simulink model "sm_car_display_battery_model"  (R2021a)
settings: Solver=VariableStepAuto  StartTime=0.0  StopTime=10.0  RelTol=1e-3
undefined symbols (not defined in the file or in its folder): X, Y, Z
libraries: sm_lib x98, nesl_utility x72, Cooling_Components x1
(part 2 of 4)

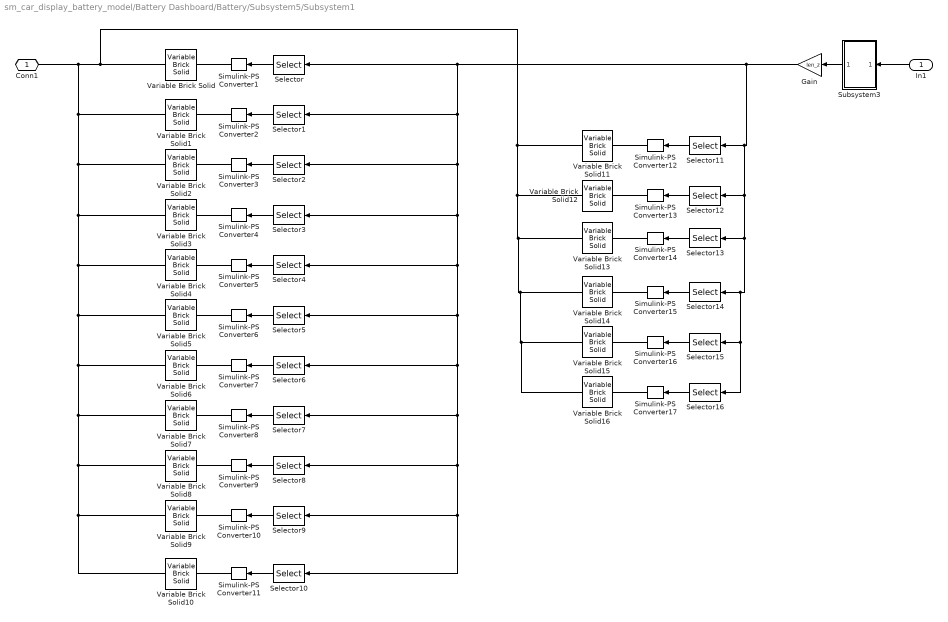
== system sm_car_display_battery_model/Battery Dashboard/Battery/Subsystem5/Subsystem1 ==
  In1 : Inport
  Gain : Gain  Gain=len_z
  Selector : Selector  InputPortWidth=numincr  IndexOptions=Index vector (dialog)  Indices=[1]  OutputSizes=1
  Selector1 : Selector  InputPortWidth=numincr  IndexOptions=Index vector (dialog)  Indices=[2]  OutputSizes=1
  Selector10 : Selector  InputPortWidth=numincr  IndexOptions=Index vector (dialog)  Indices=[11]  OutputSizes=1
  Selector11 : Selector  InputPortWidth=numincr  IndexOptions=Index vector (dialog)  Indices=[12]  OutputSizes=1
  Selector12 : Selector  InputPortWidth=numincr  IndexOptions=Index vector (dialog)  Indices=[13]  OutputSizes=1
  Selector13 : Selector  InputPortWidth=numincr  IndexOptions=Index vector (dialog)  Indices=[14]  OutputSizes=1
  Selector14 : Selector  InputPortWidth=numincr  IndexOptions=Index vector (dialog)  Indices=[15]  OutputSizes=1
  Selector15 : Selector  InputPortWidth=numincr  IndexOptions=Index vector (dialog)  Indices=[16]  OutputSizes=1
  Selector16 : Selector  InputPortWidth=numincr  IndexOptions=Index vector (dialog)  Indices=[17]  OutputSizes=1
  Selector2 : Selector  InputPortWidth=numincr  IndexOptions=Index vector (dialog)  Indices=[3]  OutputSizes=1
  Selector3 : Selector  InputPortWidth=numincr  IndexOptions=Index vector (dialog)  Indices=[4]  OutputSizes=1
  Selector4 : Selector  InputPortWidth=numincr  IndexOptions=Index vector (dialog)  Indices=[5]  OutputSizes=1
  Selector5 : Selector  InputPortWidth=numincr  IndexOptions=Index vector (dialog)  Indices=[6]  OutputSizes=1
  Selector6 : Selector  InputPortWidth=numincr  IndexOptions=Index vector (dialog)  Indices=[7]  OutputSizes=1
  Selector7 : Selector  InputPortWidth=numincr  IndexOptions=Index vector (dialog)  Indices=[8]  OutputSizes=1
  Selector8 : Selector  InputPortWidth=numincr  IndexOptions=Index vector (dialog)  Indices=[9]  OutputSizes=1
  Selector9 : Selector  InputPortWidth=numincr  IndexOptions=Index vector (dialog)  Indices=[10]  OutputSizes=1
  Simulink-PS Converter{1..17} (17 alike) : nesl_utility/Simulink-PS Converter  PhysicalDomain=network_engine_domain  SubClassName=ps_input  LeftPortType=input  RightPortType=output  PseudoPeriodic=off  Frequencies=[]  NoiseDistribution=none  NoiseParameters=[]  Unit=m  AffineConversion=off  FilteringAndDerivatives=provide  SimscapeFilterOrder=1  InputFilterTimeConstant=0.001  UdotUserProvided=0
      settings: SourceProductBaseCode=PW,SS
  Subsystem3 : Subsystem
  Variable Brick Solid : sm_lib/Body Elements/Variable Mass/Variable Brick Solid  XLengthType=Constant  XLength=len_x  XLengthUnits=m  YLengthType=Constant  YLength=len_y  YLengthUnits=m  ZLengthType=ProvidedByInput  ZLength=1  ZLengthUnits=m  MassType=CalculateFromGeometry  InitialMassType=Specified  InitialMass=1  InitialMassUnits=kg  Density=0.001  DensityUnits=kg/m^3  SenseXLength=off  SenseYLength=off  SenseZLength=off  SenseMass=off  SenseCenterOfMass=off  SenseInertiaMatrix=off  GraphicType=FromGeometry  MarkerShape=Sphere  MarkerSize=10  GraphicVisPropType=SimpleVisualProperties  GraphicDiffuseColor=[clr1]*17/numincr+[clr2]*0/numincr  GraphicSpecularColor=[0.5 0.5 0.5 1.0]  GraphicAmbientColor=[0.15 0.15 0.15 1.0]  GraphicEmissiveColor=[0.0 0.0 0.0 1.0]  GraphicShininess=75  GraphicOpacity=1.0
      settings: AttributesFormatString=%<GraphicDiffuseColor>  SourceProductBaseCode=MS
  Variable Brick Solid1 : sm_lib/Body Elements/Variable Mass/Variable Brick Solid  XLengthType=Constant  XLength=len_x  XLengthUnits=m  YLengthType=Constant  YLength=len_y  YLengthUnits=m  ZLengthType=ProvidedByInput  ZLength=1  ZLengthUnits=m  MassType=CalculateFromGeometry  InitialMassType=Specified  InitialMass=1  InitialMassUnits=kg  Density=0.001  DensityUnits=kg/m^3  SenseXLength=off  SenseYLength=off  SenseZLength=off  SenseMass=off  SenseCenterOfMass=off  SenseInertiaMatrix=off  GraphicType=FromGeometry  MarkerShape=Sphere  MarkerSize=10  GraphicVisPropType=SimpleVisualProperties  GraphicDiffuseColor=[clr1]*16/numincr+[clr2]*1/numincr  GraphicSpecularColor=[0.5 0.5 0.5 1.0]  GraphicAmbientColor=[0.15 0.15 0.15 1.0]  GraphicEmissiveColor=[0.0 0.0 0.0 1.0]  GraphicShininess=75  GraphicOpacity=1.0
      settings: AttributesFormatString=%<GraphicDiffuseColor>  SourceProductBaseCode=MS
  Variable Brick Solid10 : sm_lib/Body Elements/Variable Mass/Variable Brick Solid  XLengthType=Constant  XLength=len_x  XLengthUnits=m  YLengthType=Constant  YLength=len_y  YLengthUnits=m  ZLengthType=ProvidedByInput  ZLength=1  ZLengthUnits=m  MassType=CalculateFromGeometry  InitialMassType=Specified  InitialMass=1  InitialMassUnits=kg  Density=0.001  DensityUnits=kg/m^3  SenseXLength=off  SenseYLength=off  SenseZLength=off  SenseMass=off  SenseCenterOfMass=off  SenseInertiaMatrix=off  GraphicType=FromGeometry  MarkerShape=Sphere  MarkerSize=10  GraphicVisPropType=SimpleVisualProperties  GraphicDiffuseColor=[clr1]*7/numincr+[clr2]*10/numincr  GraphicSpecularColor=[0.5 0.5 0.5 1.0]  GraphicAmbientColor=[0.15 0.15 0.15 1.0]  GraphicEmissiveColor=[0.0 0.0 0.0 1.0]  GraphicShininess=75  GraphicOpacity=1.0
      settings: AttributesFormatString=%<GraphicDiffuseColor>  SourceProductBaseCode=MS
  Variable Brick Solid11 : sm_lib/Body Elements/Variable Mass/Variable Brick Solid  XLengthType=Constant  XLength=len_x  XLengthUnits=m  YLengthType=Constant  YLength=len_y  YLengthUnits=m  ZLengthType=ProvidedByInput  ZLength=1  ZLengthUnits=m  MassType=CalculateFromGeometry  InitialMassType=Specified  InitialMass=1  InitialMassUnits=kg  Density=0.001  DensityUnits=kg/m^3  SenseXLength=off  SenseYLength=off  SenseZLength=off  SenseMass=off  SenseCenterOfMass=off  SenseInertiaMatrix=off  GraphicType=FromGeometry  MarkerShape=Sphere  MarkerSize=10  GraphicVisPropType=SimpleVisualProperties  GraphicDiffuseColor=[clr1]*6/numincr+[clr2]*11/numincr  GraphicSpecularColor=[0.5 0.5 0.5 1.0]  GraphicAmbientColor=[0.15 0.15 0.15 1.0]  GraphicEmissiveColor=[0.0 0.0 0.0 1.0]  GraphicShininess=75  GraphicOpacity=1.0
      settings: AttributesFormatString=%<GraphicDiffuseColor>  SourceProductBaseCode=MS
  Variable Brick Solid12 : sm_lib/Body Elements/Variable Mass/Variable Brick Solid  XLengthType=Constant  XLength=len_x  XLengthUnits=m  YLengthType=Constant  YLength=len_y  YLengthUnits=m  ZLengthType=ProvidedByInput  ZLength=1  ZLengthUnits=m  MassType=CalculateFromGeometry  InitialMassType=Specified  InitialMass=1  InitialMassUnits=kg  Density=0.001  DensityUnits=kg/m^3  SenseXLength=off  SenseYLength=off  SenseZLength=off  SenseMass=off  SenseCenterOfMass=off  SenseInertiaMatrix=off  GraphicType=FromGeometry  MarkerShape=Sphere  MarkerSize=10  GraphicVisPropType=SimpleVisualProperties  GraphicDiffuseColor=[clr1]*5/numincr+[clr2]*12/numincr  GraphicSpecularColor=[0.5 0.5 0.5 1.0]  GraphicAmbientColor=[0.15 0.15 0.15 1.0]  GraphicEmissiveColor=[0.0 0.0 0.0 1.0]  GraphicShininess=75  GraphicOpacity=1.0
      settings: AttributesFormatString=%<GraphicDiffuseColor>  SourceProductBaseCode=MS
  Variable Brick Solid13 : sm_lib/Body Elements/Variable Mass/Variable Brick Solid  XLengthType=Constant  XLength=len_x  XLengthUnits=m  YLengthType=Constant  YLength=len_y  YLengthUnits=m  ZLengthType=ProvidedByInput  ZLength=1  ZLengthUnits=m  MassType=CalculateFromGeometry  InitialMassType=Specified  InitialMass=1  InitialMassUnits=kg  Density=0.001  DensityUnits=kg/m^3  SenseXLength=off  SenseYLength=off  SenseZLength=off  SenseMass=off  SenseCenterOfMass=off  SenseInertiaMatrix=off  GraphicType=FromGeometry  MarkerShape=Sphere  MarkerSize=10  GraphicVisPropType=SimpleVisualProperties  GraphicDiffuseColor=[clr1]*4/numincr+[clr2]*13/numincr  GraphicSpecularColor=[0.5 0.5 0.5 1.0]  GraphicAmbientColor=[0.15 0.15 0.15 1.0]  GraphicEmissiveColor=[0.0 0.0 0.0 1.0]  GraphicShininess=75  GraphicOpacity=1.0
      settings: AttributesFormatString=%<GraphicDiffuseColor>  SourceProductBaseCode=MS
  Variable Brick Solid14 : sm_lib/Body Elements/Variable Mass/Variable Brick Solid  XLengthType=Constant  XLength=len_x  XLengthUnits=m  YLengthType=Constant  YLength=len_y  YLengthUnits=m  ZLengthType=ProvidedByInput  ZLength=1  ZLengthUnits=m  MassType=CalculateFromGeometry  InitialMassType=Specified  InitialMass=1  InitialMassUnits=kg  Density=0.001  DensityUnits=kg/m^3  SenseXLength=off  SenseYLength=off  SenseZLength=off  SenseMass=off  SenseCenterOfMass=off  SenseInertiaMatrix=off  GraphicType=FromGeometry  MarkerShape=Sphere  MarkerSize=10  GraphicVisPropType=SimpleVisualProperties  GraphicDiffuseColor=[clr1]*3/numincr+[clr2]*14/numincr  GraphicSpecularColor=[0.5 0.5 0.5 1.0]  GraphicAmbientColor=[0.15 0.15 0.15 1.0]  GraphicEmissiveColor=[0.0 0.0 0.0 1.0]  GraphicShininess=75  GraphicOpacity=1.0
      settings: AttributesFormatString=%<GraphicDiffuseColor>  SourceProductBaseCode=MS
  Variable Brick Solid15 : sm_lib/Body Elements/Variable Mass/Variable Brick Solid  XLengthType=Constant  XLength=len_x  XLengthUnits=m  YLengthType=Constant  YLength=len_y  YLengthUnits=m  ZLengthType=ProvidedByInput  ZLength=1  ZLengthUnits=m  MassType=CalculateFromGeometry  InitialMassType=Specified  InitialMass=1  InitialMassUnits=kg  Density=0.001  DensityUnits=kg/m^3  SenseXLength=off  SenseYLength=off  SenseZLength=off  SenseMass=off  SenseCenterOfMass=off  SenseInertiaMatrix=off  GraphicType=FromGeometry  MarkerShape=Sphere  MarkerSize=10  GraphicVisPropType=SimpleVisualProperties  GraphicDiffuseColor=[clr1]*2/numincr+[clr2]*15/numincr  GraphicSpecularColor=[0.5 0.5 0.5 1.0]  GraphicAmbientColor=[0.15 0.15 0.15 1.0]  GraphicEmissiveColor=[0.0 0.0 0.0 1.0]  GraphicShininess=75  GraphicOpacity=1.0
      settings: AttributesFormatString=%<GraphicDiffuseColor>  SourceProductBaseCode=MS
  Variable Brick Solid16 : sm_lib/Body Elements/Variable Mass/Variable Brick Solid  XLengthType=Constant  XLength=len_x  XLengthUnits=m  YLengthType=Constant  YLength=len_y  YLengthUnits=m  ZLengthType=ProvidedByInput  ZLength=1  ZLengthUnits=m  MassType=CalculateFromGeometry  InitialMassType=Specified  InitialMass=1  InitialMassUnits=kg  Density=0.001  DensityUnits=kg/m^3  SenseXLength=off  SenseYLength=off  SenseZLength=off  SenseMass=off  SenseCenterOfMass=off  SenseInertiaMatrix=off  GraphicType=FromGeometry  MarkerShape=Sphere  MarkerSize=10  GraphicVisPropType=SimpleVisualProperties  GraphicDiffuseColor=[clr1]*1/numincr+[clr2]*16/numincr  GraphicSpecularColor=[0.5 0.5 0.5 1.0]  GraphicAmbientColor=[0.15 0.15 0.15 1.0]  GraphicEmissiveColor=[0.0 0.0 0.0 1.0]  GraphicShininess=75  GraphicOpacity=1.0
      settings: AttributesFormatString=%<GraphicDiffuseColor>  SourceProductBaseCode=MS
  Variable Brick Solid2 : sm_lib/Body Elements/Variable Mass/Variable Brick Solid  XLengthType=Constant  XLength=len_x  XLengthUnits=m  YLengthType=Constant  YLength=len_y  YLengthUnits=m  ZLengthType=ProvidedByInput  ZLength=1  ZLengthUnits=m  MassType=CalculateFromGeometry  InitialMassType=Specified  InitialMass=1  InitialMassUnits=kg  Density=0.001  DensityUnits=kg/m^3  SenseXLength=off  SenseYLength=off  SenseZLength=off  SenseMass=off  SenseCenterOfMass=off  SenseInertiaMatrix=off  GraphicType=FromGeometry  MarkerShape=Sphere  MarkerSize=10  GraphicVisPropType=SimpleVisualProperties  GraphicDiffuseColor=[clr1]*15/numincr+[clr2]*2/numincr  GraphicSpecularColor=[0.5 0.5 0.5 1.0]  GraphicAmbientColor=[0.15 0.15 0.15 1.0]  GraphicEmissiveColor=[0.0 0.0 0.0 1.0]  GraphicShininess=75  GraphicOpacity=1.0
      settings: AttributesFormatString=%<GraphicDiffuseColor>  SourceProductBaseCode=MS
  Variable Brick Solid3 : sm_lib/Body Elements/Variable Mass/Variable Brick Solid  XLengthType=Constant  XLength=len_x  XLengthUnits=m  YLengthType=Constant  YLength=len_y  YLengthUnits=m  ZLengthType=ProvidedByInput  ZLength=1  ZLengthUnits=m  MassType=CalculateFromGeometry  InitialMassType=Specified  InitialMass=1  InitialMassUnits=kg  Density=0.001  DensityUnits=kg/m^3  SenseXLength=off  SenseYLength=off  SenseZLength=off  SenseMass=off  SenseCenterOfMass=off  SenseInertiaMatrix=off  GraphicType=FromGeometry  MarkerShape=Sphere  MarkerSize=10  GraphicVisPropType=SimpleVisualProperties  GraphicDiffuseColor=[clr1]*14/numincr+[clr2]*3/numincr  GraphicSpecularColor=[0.5 0.5 0.5 1.0]  GraphicAmbientColor=[0.15 0.15 0.15 1.0]  GraphicEmissiveColor=[0.0 0.0 0.0 1.0]  GraphicShininess=75  GraphicOpacity=1.0
      settings: AttributesFormatString=%<GraphicDiffuseColor>  SourceProductBaseCode=MS
  Variable Brick Solid4 : sm_lib/Body Elements/Variable Mass/Variable Brick Solid  XLengthType=Constant  XLength=len_x  XLengthUnits=m  YLengthType=Constant  YLength=len_y  YLengthUnits=m  ZLengthType=ProvidedByInput  ZLength=1  ZLengthUnits=m  MassType=CalculateFromGeometry  InitialMassType=Specified  InitialMass=1  InitialMassUnits=kg  Density=0.001  DensityUnits=kg/m^3  SenseXLength=off  SenseYLength=off  SenseZLength=off  SenseMass=off  SenseCenterOfMass=off  SenseInertiaMatrix=off  GraphicType=FromGeometry  MarkerShape=Sphere  MarkerSize=10  GraphicVisPropType=SimpleVisualProperties  GraphicDiffuseColor=[clr1]*13/numincr+[clr2]*4/numincr  GraphicSpecularColor=[0.5 0.5 0.5 1.0]  GraphicAmbientColor=[0.15 0.15 0.15 1.0]  GraphicEmissiveColor=[0.0 0.0 0.0 1.0]  GraphicShininess=75  GraphicOpacity=1.0
      settings: AttributesFormatString=%<GraphicDiffuseColor>  SourceProductBaseCode=MS
  Variable Brick Solid5 : sm_lib/Body Elements/Variable Mass/Variable Brick Solid  XLengthType=Constant  XLength=len_x  XLengthUnits=m  YLengthType=Constant  YLength=len_y  YLengthUnits=m  ZLengthType=ProvidedByInput  ZLength=1  ZLengthUnits=m  MassType=CalculateFromGeometry  InitialMassType=Specified  InitialMass=1  InitialMassUnits=kg  Density=0.001  DensityUnits=kg/m^3  SenseXLength=off  SenseYLength=off  SenseZLength=off  SenseMass=off  SenseCenterOfMass=off  SenseInertiaMatrix=off  GraphicType=FromGeometry  MarkerShape=Sphere  MarkerSize=10  GraphicVisPropType=SimpleVisualProperties  GraphicDiffuseColor=[clr1]*12/numincr+[clr2]*5/numincr  GraphicSpecularColor=[0.5 0.5 0.5 1.0]  GraphicAmbientColor=[0.15 0.15 0.15 1.0]  GraphicEmissiveColor=[0.0 0.0 0.0 1.0]  GraphicShininess=75  GraphicOpacity=1.0
      settings: AttributesFormatString=%<GraphicDiffuseColor>  SourceProductBaseCode=MS
  Variable Brick Solid6 : sm_lib/Body Elements/Variable Mass/Variable Brick Solid  XLengthType=Constant  XLength=len_x  XLengthUnits=m  YLengthType=Constant  YLength=len_y  YLengthUnits=m  ZLengthType=ProvidedByInput  ZLength=1  ZLengthUnits=m  MassType=CalculateFromGeometry  InitialMassType=Specified  InitialMass=1  InitialMassUnits=kg  Density=0.001  DensityUnits=kg/m^3  SenseXLength=off  SenseYLength=off  SenseZLength=off  SenseMass=off  SenseCenterOfMass=off  SenseInertiaMatrix=off  GraphicType=FromGeometry  MarkerShape=Sphere  MarkerSize=10  GraphicVisPropType=SimpleVisualProperties  GraphicDiffuseColor=[clr1]*11/numincr+[clr2]*6/numincr  GraphicSpecularColor=[0.5 0.5 0.5 1.0]  GraphicAmbientColor=[0.15 0.15 0.15 1.0]  GraphicEmissiveColor=[0.0 0.0 0.0 1.0]  GraphicShininess=75  GraphicOpacity=1.0
      settings: AttributesFormatString=%<GraphicDiffuseColor>  SourceProductBaseCode=MS
  Variable Brick Solid7 : sm_lib/Body Elements/Variable Mass/Variable Brick Solid  XLengthType=Constant  XLength=len_x  XLengthUnits=m  YLengthType=Constant  YLength=len_y  YLengthUnits=m  ZLengthType=ProvidedByInput  ZLength=1  ZLengthUnits=m  MassType=CalculateFromGeometry  InitialMassType=Specified  InitialMass=1  InitialMassUnits=kg  Density=0.001  DensityUnits=kg/m^3  SenseXLength=off  SenseYLength=off  SenseZLength=off  SenseMass=off  SenseCenterOfMass=off  SenseInertiaMatrix=off  GraphicType=FromGeometry  MarkerShape=Sphere  MarkerSize=10  GraphicVisPropType=SimpleVisualProperties  GraphicDiffuseColor=[clr1]*10/numincr+[clr2]*7/numincr  GraphicSpecularColor=[0.5 0.5 0.5 1.0]  GraphicAmbientColor=[0.15 0.15 0.15 1.0]  GraphicEmissiveColor=[0.0 0.0 0.0 1.0]  GraphicShininess=75  GraphicOpacity=1.0
      settings: AttributesFormatString=%<GraphicDiffuseColor>  SourceProductBaseCode=MS
  Variable Brick Solid8 : sm_lib/Body Elements/Variable Mass/Variable Brick Solid  XLengthType=Constant  XLength=len_x  XLengthUnits=m  YLengthType=Constant  YLength=len_y  YLengthUnits=m  ZLengthType=ProvidedByInput  ZLength=1  ZLengthUnits=m  MassType=CalculateFromGeometry  InitialMassType=Specified  InitialMass=1  InitialMassUnits=kg  Density=0.001  DensityUnits=kg/m^3  SenseXLength=off  SenseYLength=off  SenseZLength=off  SenseMass=off  SenseCenterOfMass=off  SenseInertiaMatrix=off  GraphicType=FromGeometry  MarkerShape=Sphere  MarkerSize=10  GraphicVisPropType=SimpleVisualProperties  GraphicDiffuseColor=[clr1]*9/numincr+[clr2]*8/numincr  GraphicSpecularColor=[0.5 0.5 0.5 1.0]  GraphicAmbientColor=[0.15 0.15 0.15 1.0]  GraphicEmissiveColor=[0.0 0.0 0.0 1.0]  GraphicShininess=75  GraphicOpacity=1.0
      settings: AttributesFormatString=%<GraphicDiffuseColor>  SourceProductBaseCode=MS
  Variable Brick Solid9 : sm_lib/Body Elements/Variable Mass/Variable Brick Solid  XLengthType=Constant  XLength=len_x  XLengthUnits=m  YLengthType=Constant  YLength=len_y  YLengthUnits=m  ZLengthType=ProvidedByInput  ZLength=1  ZLengthUnits=m  MassType=CalculateFromGeometry  InitialMassType=Specified  InitialMass=1  InitialMassUnits=kg  Density=0.001  DensityUnits=kg/m^3  SenseXLength=off  SenseYLength=off  SenseZLength=off  SenseMass=off  SenseCenterOfMass=off  SenseInertiaMatrix=off  GraphicType=FromGeometry  MarkerShape=Sphere  MarkerSize=10  GraphicVisPropType=SimpleVisualProperties  GraphicDiffuseColor=[clr1]*8/numincr+[clr2]*9/numincr  GraphicSpecularColor=[0.5 0.5 0.5 1.0]  GraphicAmbientColor=[0.15 0.15 0.15 1.0]  GraphicEmissiveColor=[0.0 0.0 0.0 1.0]  GraphicShininess=75  GraphicOpacity=1.0
      settings: AttributesFormatString=%<GraphicDiffuseColor>  SourceProductBaseCode=MS
  Conn1 : PMIOPort  Side=Right
  wires:
  Selector/1 -> Simulink-PS Converter1/1
  Selector1/1 -> Simulink-PS Converter2/1
  Selector2/1 -> Simulink-PS Converter3/1
  Selector3/1 -> Simulink-PS Converter4/1
  Selector4/1 -> Simulink-PS Converter5/1
  Selector5/1 -> Simulink-PS Converter6/1
  Selector6/1 -> Simulink-PS Converter7/1
  Selector7/1 -> Simulink-PS Converter8/1
  Selector8/1 -> Simulink-PS Converter9/1
  Selector9/1 -> Simulink-PS Converter10/1
  Selector10/1 -> Simulink-PS Converter11/1
  Selector11/1 -> Simulink-PS Converter12/1
  Selector12/1 -> Simulink-PS Converter13/1
  Selector13/1 -> Simulink-PS Converter14/1
  Selector14/1 -> Simulink-PS Converter15/1
  Selector15/1 -> Simulink-PS Converter16/1
  In1/1 -> Subsystem3/1(In1)
  Selector16/1 -> Simulink-PS Converter17/1
  Gain/1 -> Selector16/1, Selector15/1, Selector14/1, Selector13/1, Selector12/1, Selector11/1, Selector10/1, Selector9/1, Selector8/1, Selector7/1, Selector6/1, Selector5/1, Selector4/1, Selector3/1, Selector2/1, Selector1/1, Selector/1
  Subsystem3/1(Out1) -> Gain/1
  connections:
  Simulink-PS Converter1/RConn1 -- Variable Brick Solid/LConn1
  Variable Brick Solid12/RConn1 -- Variable Brick Solid1/RConn1 -- Variable Brick Solid2/RConn1 -- Variable Brick Solid3/RConn1 -- Variable Brick Solid5/RConn1 -- Variable Brick Solid6/RConn1 -- Variable Brick Solid7/RConn1 -- Variable Brick Solid8/RConn1 -- Variable Brick Solid9/RConn1 -- Variable Brick Solid10/RConn1 -- Variable Brick Solid4/RConn1 -- Conn1/RConn1 -- Variable Brick Solid/RConn1 -- Variable Brick Solid11/RConn1 -- Variable Brick Solid13/RConn1 -- Variable Brick Solid14/RConn1 -- Variable Brick Solid15/RConn1 -- Variable Brick Solid16/RConn1
  Simulink-PS Converter2/RConn1 -- Variable Brick Solid1/LConn1
  Variable Brick Solid2/LConn1 -- Simulink-PS Converter3/RConn1
  Variable Brick Solid3/LConn1 -- Simulink-PS Converter4/RConn1
  Variable Brick Solid4/LConn1 -- Simulink-PS Converter5/RConn1
  Variable Brick Solid5/LConn1 -- Simulink-PS Converter6/RConn1
  Variable Brick Solid6/LConn1 -- Simulink-PS Converter7/RConn1
  Variable Brick Solid7/LConn1 -- Simulink-PS Converter8/RConn1
  Variable Brick Solid8/LConn1 -- Simulink-PS Converter9/RConn1
  Variable Brick Solid9/LConn1 -- Simulink-PS Converter10/RConn1
  Variable Brick Solid10/LConn1 -- Simulink-PS Converter11/RConn1
  Variable Brick Solid11/LConn1 -- Simulink-PS Converter12/RConn1
  Variable Brick Solid12/LConn1 -- Simulink-PS Converter13/RConn1
  Variable Brick Solid13/LConn1 -- Simulink-PS Converter14/RConn1
  Variable Brick Solid14/LConn1 -- Simulink-PS Converter15/RConn1
  Variable Brick Solid15/LConn1 -- Simulink-PS Converter16/RConn1
  Variable Brick Solid16/LConn1 -- Simulink-PS Converter17/RConn1

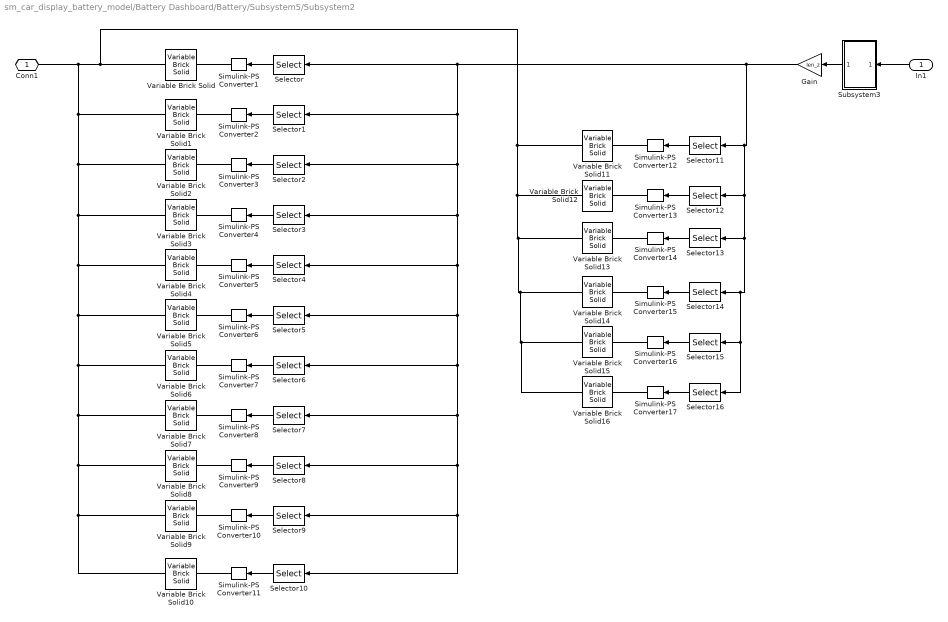
== system sm_car_display_battery_model/Battery Dashboard/Battery/Subsystem5/Subsystem2 ==
  In1 : Inport
  Gain : Gain  Gain=len_z
  Selector : Selector  InputPortWidth=numincr  IndexOptions=Index vector (dialog)  Indices=[1]  OutputSizes=1
  Selector1 : Selector  InputPortWidth=numincr  IndexOptions=Index vector (dialog)  Indices=[2]  OutputSizes=1
  Selector10 : Selector  InputPortWidth=numincr  IndexOptions=Index vector (dialog)  Indices=[11]  OutputSizes=1
  Selector11 : Selector  InputPortWidth=numincr  IndexOptions=Index vector (dialog)  Indices=[12]  OutputSizes=1
  Selector12 : Selector  InputPortWidth=numincr  IndexOptions=Index vector (dialog)  Indices=[13]  OutputSizes=1
  Selector13 : Selector  InputPortWidth=numincr  IndexOptions=Index vector (dialog)  Indices=[14]  OutputSizes=1
  Selector14 : Selector  InputPortWidth=numincr  IndexOptions=Index vector (dialog)  Indices=[15]  OutputSizes=1
  Selector15 : Selector  InputPortWidth=numincr  IndexOptions=Index vector (dialog)  Indices=[16]  OutputSizes=1
  Selector16 : Selector  InputPortWidth=numincr  IndexOptions=Index vector (dialog)  Indices=[17]  OutputSizes=1
  Selector2 : Selector  InputPortWidth=numincr  IndexOptions=Index vector (dialog)  Indices=[3]  OutputSizes=1
  Selector3 : Selector  InputPortWidth=numincr  IndexOptions=Index vector (dialog)  Indices=[4]  OutputSizes=1
  Selector4 : Selector  InputPortWidth=numincr  IndexOptions=Index vector (dialog)  Indices=[5]  OutputSizes=1
  Selector5 : Selector  InputPortWidth=numincr  IndexOptions=Index vector (dialog)  Indices=[6]  OutputSizes=1
  Selector6 : Selector  InputPortWidth=numincr  IndexOptions=Index vector (dialog)  Indices=[7]  OutputSizes=1
  Selector7 : Selector  InputPortWidth=numincr  IndexOptions=Index vector (dialog)  Indices=[8]  OutputSizes=1
  Selector8 : Selector  InputPortWidth=numincr  IndexOptions=Index vector (dialog)  Indices=[9]  OutputSizes=1
  Selector9 : Selector  InputPortWidth=numincr  IndexOptions=Index vector (dialog)  Indices=[10]  OutputSizes=1
  Simulink-PS Converter{1..17} (17 alike) : nesl_utility/Simulink-PS Converter  PhysicalDomain=network_engine_domain  SubClassName=ps_input  LeftPortType=input  RightPortType=output  PseudoPeriodic=off  Frequencies=[]  NoiseDistribution=none  NoiseParameters=[]  Unit=m  AffineConversion=off  FilteringAndDerivatives=provide  SimscapeFilterOrder=1  InputFilterTimeConstant=0.001  UdotUserProvided=0
      settings: SourceProductBaseCode=PW,SS
  Subsystem3 : Subsystem
  Variable Brick Solid : sm_lib/Body Elements/Variable Mass/Variable Brick Solid  XLengthType=Constant  XLength=len_x  XLengthUnits=m  YLengthType=Constant  YLength=len_y  YLengthUnits=m  ZLengthType=ProvidedByInput  ZLength=1  ZLengthUnits=m  MassType=CalculateFromGeometry  InitialMassType=Specified  InitialMass=1  InitialMassUnits=kg  Density=0.001  DensityUnits=kg/m^3  SenseXLength=off  SenseYLength=off  SenseZLength=off  SenseMass=off  SenseCenterOfMass=off  SenseInertiaMatrix=off  GraphicType=FromGeometry  MarkerShape=Sphere  MarkerSize=10  GraphicVisPropType=SimpleVisualProperties  GraphicDiffuseColor=[clr1]*17/numincr+[clr2]*0/numincr  GraphicSpecularColor=[0.5 0.5 0.5 1.0]  GraphicAmbientColor=[0.15 0.15 0.15 1.0]  GraphicEmissiveColor=[0.0 0.0 0.0 1.0]  GraphicShininess=75  GraphicOpacity=1.0
      settings: AttributesFormatString=%<GraphicDiffuseColor>  SourceProductBaseCode=MS
  Variable Brick Solid1 : sm_lib/Body Elements/Variable Mass/Variable Brick Solid  XLengthType=Constant  XLength=len_x  XLengthUnits=m  YLengthType=Constant  YLength=len_y  YLengthUnits=m  ZLengthType=ProvidedByInput  ZLength=1  ZLengthUnits=m  MassType=CalculateFromGeometry  InitialMassType=Specified  InitialMass=1  InitialMassUnits=kg  Density=0.001  DensityUnits=kg/m^3  SenseXLength=off  SenseYLength=off  SenseZLength=off  SenseMass=off  SenseCenterOfMass=off  SenseInertiaMatrix=off  GraphicType=FromGeometry  MarkerShape=Sphere  MarkerSize=10  GraphicVisPropType=SimpleVisualProperties  GraphicDiffuseColor=[clr1]*16/numincr+[clr2]*1/numincr  GraphicSpecularColor=[0.5 0.5 0.5 1.0]  GraphicAmbientColor=[0.15 0.15 0.15 1.0]  GraphicEmissiveColor=[0.0 0.0 0.0 1.0]  GraphicShininess=75  GraphicOpacity=1.0
      settings: AttributesFormatString=%<GraphicDiffuseColor>  SourceProductBaseCode=MS
  Variable Brick Solid10 : sm_lib/Body Elements/Variable Mass/Variable Brick Solid  XLengthType=Constant  XLength=len_x  XLengthUnits=m  YLengthType=Constant  YLength=len_y  YLengthUnits=m  ZLengthType=ProvidedByInput  ZLength=1  ZLengthUnits=m  MassType=CalculateFromGeometry  InitialMassType=Specified  InitialMass=1  InitialMassUnits=kg  Density=0.001  DensityUnits=kg/m^3  SenseXLength=off  SenseYLength=off  SenseZLength=off  SenseMass=off  SenseCenterOfMass=off  SenseInertiaMatrix=off  GraphicType=FromGeometry  MarkerShape=Sphere  MarkerSize=10  GraphicVisPropType=SimpleVisualProperties  GraphicDiffuseColor=[clr1]*7/numincr+[clr2]*10/numincr  GraphicSpecularColor=[0.5 0.5 0.5 1.0]  GraphicAmbientColor=[0.15 0.15 0.15 1.0]  GraphicEmissiveColor=[0.0 0.0 0.0 1.0]  GraphicShininess=75  GraphicOpacity=1.0
      settings: AttributesFormatString=%<GraphicDiffuseColor>  SourceProductBaseCode=MS
  Variable Brick Solid11 : sm_lib/Body Elements/Variable Mass/Variable Brick Solid  XLengthType=Constant  XLength=len_x  XLengthUnits=m  YLengthType=Constant  YLength=len_y  YLengthUnits=m  ZLengthType=ProvidedByInput  ZLength=1  ZLengthUnits=m  MassType=CalculateFromGeometry  InitialMassType=Specified  InitialMass=1  InitialMassUnits=kg  Density=0.001  DensityUnits=kg/m^3  SenseXLength=off  SenseYLength=off  SenseZLength=off  SenseMass=off  SenseCenterOfMass=off  SenseInertiaMatrix=off  GraphicType=FromGeometry  MarkerShape=Sphere  MarkerSize=10  GraphicVisPropType=SimpleVisualProperties  GraphicDiffuseColor=[clr1]*6/numincr+[clr2]*11/numincr  GraphicSpecularColor=[0.5 0.5 0.5 1.0]  GraphicAmbientColor=[0.15 0.15 0.15 1.0]  GraphicEmissiveColor=[0.0 0.0 0.0 1.0]  GraphicShininess=75  GraphicOpacity=1.0
      settings: AttributesFormatString=%<GraphicDiffuseColor>  SourceProductBaseCode=MS
  Variable Brick Solid12 : sm_lib/Body Elements/Variable Mass/Variable Brick Solid  XLengthType=Constant  XLength=len_x  XLengthUnits=m  YLengthType=Constant  YLength=len_y  YLengthUnits=m  ZLengthType=ProvidedByInput  ZLength=1  ZLengthUnits=m  MassType=CalculateFromGeometry  InitialMassType=Specified  InitialMass=1  InitialMassUnits=kg  Density=0.001  DensityUnits=kg/m^3  SenseXLength=off  SenseYLength=off  SenseZLength=off  SenseMass=off  SenseCenterOfMass=off  SenseInertiaMatrix=off  GraphicType=FromGeometry  MarkerShape=Sphere  MarkerSize=10  GraphicVisPropType=SimpleVisualProperties  GraphicDiffuseColor=[clr1]*5/numincr+[clr2]*12/numincr  GraphicSpecularColor=[0.5 0.5 0.5 1.0]  GraphicAmbientColor=[0.15 0.15 0.15 1.0]  GraphicEmissiveColor=[0.0 0.0 0.0 1.0]  GraphicShininess=75  GraphicOpacity=1.0
      settings: AttributesFormatString=%<GraphicDiffuseColor>  SourceProductBaseCode=MS
  Variable Brick Solid13 : sm_lib/Body Elements/Variable Mass/Variable Brick Solid  XLengthType=Constant  XLength=len_x  XLengthUnits=m  YLengthType=Constant  YLength=len_y  YLengthUnits=m  ZLengthType=ProvidedByInput  ZLength=1  ZLengthUnits=m  MassType=CalculateFromGeometry  InitialMassType=Specified  InitialMass=1  InitialMassUnits=kg  Density=0.001  DensityUnits=kg/m^3  SenseXLength=off  SenseYLength=off  SenseZLength=off  SenseMass=off  SenseCenterOfMass=off  SenseInertiaMatrix=off  GraphicType=FromGeometry  MarkerShape=Sphere  MarkerSize=10  GraphicVisPropType=SimpleVisualProperties  GraphicDiffuseColor=[clr1]*4/numincr+[clr2]*13/numincr  GraphicSpecularColor=[0.5 0.5 0.5 1.0]  GraphicAmbientColor=[0.15 0.15 0.15 1.0]  GraphicEmissiveColor=[0.0 0.0 0.0 1.0]  GraphicShininess=75  GraphicOpacity=1.0
      settings: AttributesFormatString=%<GraphicDiffuseColor>  SourceProductBaseCode=MS
  Variable Brick Solid14 : sm_lib/Body Elements/Variable Mass/Variable Brick Solid  XLengthType=Constant  XLength=len_x  XLengthUnits=m  YLengthType=Constant  YLength=len_y  YLengthUnits=m  ZLengthType=ProvidedByInput  ZLength=1  ZLengthUnits=m  MassType=CalculateFromGeometry  InitialMassType=Specified  InitialMass=1  InitialMassUnits=kg  Density=0.001  DensityUnits=kg/m^3  SenseXLength=off  SenseYLength=off  SenseZLength=off  SenseMass=off  SenseCenterOfMass=off  SenseInertiaMatrix=off  GraphicType=FromGeometry  MarkerShape=Sphere  MarkerSize=10  GraphicVisPropType=SimpleVisualProperties  GraphicDiffuseColor=[clr1]*3/numincr+[clr2]*14/numincr  GraphicSpecularColor=[0.5 0.5 0.5 1.0]  GraphicAmbientColor=[0.15 0.15 0.15 1.0]  GraphicEmissiveColor=[0.0 0.0 0.0 1.0]  GraphicShininess=75  GraphicOpacity=1.0
      settings: AttributesFormatString=%<GraphicDiffuseColor>  SourceProductBaseCode=MS
  Variable Brick Solid15 : sm_lib/Body Elements/Variable Mass/Variable Brick Solid  XLengthType=Constant  XLength=len_x  XLengthUnits=m  YLengthType=Constant  YLength=len_y  YLengthUnits=m  ZLengthType=ProvidedByInput  ZLength=1  ZLengthUnits=m  MassType=CalculateFromGeometry  InitialMassType=Specified  InitialMass=1  InitialMassUnits=kg  Density=0.001  DensityUnits=kg/m^3  SenseXLength=off  SenseYLength=off  SenseZLength=off  SenseMass=off  SenseCenterOfMass=off  SenseInertiaMatrix=off  GraphicType=FromGeometry  MarkerShape=Sphere  MarkerSize=10  GraphicVisPropType=SimpleVisualProperties  GraphicDiffuseColor=[clr1]*2/numincr+[clr2]*15/numincr  GraphicSpecularColor=[0.5 0.5 0.5 1.0]  GraphicAmbientColor=[0.15 0.15 0.15 1.0]  GraphicEmissiveColor=[0.0 0.0 0.0 1.0]  GraphicShininess=75  GraphicOpacity=1.0
      settings: AttributesFormatString=%<GraphicDiffuseColor>  SourceProductBaseCode=MS
  Variable Brick Solid16 : sm_lib/Body Elements/Variable Mass/Variable Brick Solid  XLengthType=Constant  XLength=len_x  XLengthUnits=m  YLengthType=Constant  YLength=len_y  YLengthUnits=m  ZLengthType=ProvidedByInput  ZLength=1  ZLengthUnits=m  MassType=CalculateFromGeometry  InitialMassType=Specified  InitialMass=1  InitialMassUnits=kg  Density=0.001  DensityUnits=kg/m^3  SenseXLength=off  SenseYLength=off  SenseZLength=off  SenseMass=off  SenseCenterOfMass=off  SenseInertiaMatrix=off  GraphicType=FromGeometry  MarkerShape=Sphere  MarkerSize=10  GraphicVisPropType=SimpleVisualProperties  GraphicDiffuseColor=[clr1]*1/numincr+[clr2]*16/numincr  GraphicSpecularColor=[0.5 0.5 0.5 1.0]  GraphicAmbientColor=[0.15 0.15 0.15 1.0]  GraphicEmissiveColor=[0.0 0.0 0.0 1.0]  GraphicShininess=75  GraphicOpacity=1.0
      settings: AttributesFormatString=%<GraphicDiffuseColor>  SourceProductBaseCode=MS
  Variable Brick Solid2 : sm_lib/Body Elements/Variable Mass/Variable Brick Solid  XLengthType=Constant  XLength=len_x  XLengthUnits=m  YLengthType=Constant  YLength=len_y  YLengthUnits=m  ZLengthType=ProvidedByInput  ZLength=1  ZLengthUnits=m  MassType=CalculateFromGeometry  InitialMassType=Specified  InitialMass=1  InitialMassUnits=kg  Density=0.001  DensityUnits=kg/m^3  SenseXLength=off  SenseYLength=off  SenseZLength=off  SenseMass=off  SenseCenterOfMass=off  SenseInertiaMatrix=off  GraphicType=FromGeometry  MarkerShape=Sphere  MarkerSize=10  GraphicVisPropType=SimpleVisualProperties  GraphicDiffuseColor=[clr1]*15/numincr+[clr2]*2/numincr  GraphicSpecularColor=[0.5 0.5 0.5 1.0]  GraphicAmbientColor=[0.15 0.15 0.15 1.0]  GraphicEmissiveColor=[0.0 0.0 0.0 1.0]  GraphicShininess=75  GraphicOpacity=1.0
      settings: AttributesFormatString=%<GraphicDiffuseColor>  SourceProductBaseCode=MS
  Variable Brick Solid3 : sm_lib/Body Elements/Variable Mass/Variable Brick Solid  XLengthType=Constant  XLength=len_x  XLengthUnits=m  YLengthType=Constant  YLength=len_y  YLengthUnits=m  ZLengthType=ProvidedByInput  ZLength=1  ZLengthUnits=m  MassType=CalculateFromGeometry  InitialMassType=Specified  InitialMass=1  InitialMassUnits=kg  Density=0.001  DensityUnits=kg/m^3  SenseXLength=off  SenseYLength=off  SenseZLength=off  SenseMass=off  SenseCenterOfMass=off  SenseInertiaMatrix=off  GraphicType=FromGeometry  MarkerShape=Sphere  MarkerSize=10  GraphicVisPropType=SimpleVisualProperties  GraphicDiffuseColor=[clr1]*14/numincr+[clr2]*3/numincr  GraphicSpecularColor=[0.5 0.5 0.5 1.0]  GraphicAmbientColor=[0.15 0.15 0.15 1.0]  GraphicEmissiveColor=[0.0 0.0 0.0 1.0]  GraphicShininess=75  GraphicOpacity=1.0
      settings: AttributesFormatString=%<GraphicDiffuseColor>  SourceProductBaseCode=MS
  Variable Brick Solid4 : sm_lib/Body Elements/Variable Mass/Variable Brick Solid  XLengthType=Constant  XLength=len_x  XLengthUnits=m  YLengthType=Constant  YLength=len_y  YLengthUnits=m  ZLengthType=ProvidedByInput  ZLength=1  ZLengthUnits=m  MassType=CalculateFromGeometry  InitialMassType=Specified  InitialMass=1  InitialMassUnits=kg  Density=0.001  DensityUnits=kg/m^3  SenseXLength=off  SenseYLength=off  SenseZLength=off  SenseMass=off  SenseCenterOfMass=off  SenseInertiaMatrix=off  GraphicType=FromGeometry  MarkerShape=Sphere  MarkerSize=10  GraphicVisPropType=SimpleVisualProperties  GraphicDiffuseColor=[clr1]*13/numincr+[clr2]*4/numincr  GraphicSpecularColor=[0.5 0.5 0.5 1.0]  GraphicAmbientColor=[0.15 0.15 0.15 1.0]  GraphicEmissiveColor=[0.0 0.0 0.0 1.0]  GraphicShininess=75  GraphicOpacity=1.0
      settings: AttributesFormatString=%<GraphicDiffuseColor>  SourceProductBaseCode=MS
  Variable Brick Solid5 : sm_lib/Body Elements/Variable Mass/Variable Brick Solid  XLengthType=Constant  XLength=len_x  XLengthUnits=m  YLengthType=Constant  YLength=len_y  YLengthUnits=m  ZLengthType=ProvidedByInput  ZLength=1  ZLengthUnits=m  MassType=CalculateFromGeometry  InitialMassType=Specified  InitialMass=1  InitialMassUnits=kg  Density=0.001  DensityUnits=kg/m^3  SenseXLength=off  SenseYLength=off  SenseZLength=off  SenseMass=off  SenseCenterOfMass=off  SenseInertiaMatrix=off  GraphicType=FromGeometry  MarkerShape=Sphere  MarkerSize=10  GraphicVisPropType=SimpleVisualProperties  GraphicDiffuseColor=[clr1]*12/numincr+[clr2]*5/numincr  GraphicSpecularColor=[0.5 0.5 0.5 1.0]  GraphicAmbientColor=[0.15 0.15 0.15 1.0]  GraphicEmissiveColor=[0.0 0.0 0.0 1.0]  GraphicShininess=75  GraphicOpacity=1.0
      settings: AttributesFormatString=%<GraphicDiffuseColor>  SourceProductBaseCode=MS
  Variable Brick Solid6 : sm_lib/Body Elements/Variable Mass/Variable Brick Solid  XLengthType=Constant  XLength=len_x  XLengthUnits=m  YLengthType=Constant  YLength=len_y  YLengthUnits=m  ZLengthType=ProvidedByInput  ZLength=1  ZLengthUnits=m  MassType=CalculateFromGeometry  InitialMassType=Specified  InitialMass=1  InitialMassUnits=kg  Density=0.001  DensityUnits=kg/m^3  SenseXLength=off  SenseYLength=off  SenseZLength=off  SenseMass=off  SenseCenterOfMass=off  SenseInertiaMatrix=off  GraphicType=FromGeometry  MarkerShape=Sphere  MarkerSize=10  GraphicVisPropType=SimpleVisualProperties  GraphicDiffuseColor=[clr1]*11/numincr+[clr2]*6/numincr  GraphicSpecularColor=[0.5 0.5 0.5 1.0]  GraphicAmbientColor=[0.15 0.15 0.15 1.0]  GraphicEmissiveColor=[0.0 0.0 0.0 1.0]  GraphicShininess=75  GraphicOpacity=1.0
      settings: AttributesFormatString=%<GraphicDiffuseColor>  SourceProductBaseCode=MS
  Variable Brick Solid7 : sm_lib/Body Elements/Variable Mass/Variable Brick Solid  XLengthType=Constant  XLength=len_x  XLengthUnits=m  YLengthType=Constant  YLength=len_y  YLengthUnits=m  ZLengthType=ProvidedByInput  ZLength=1  ZLengthUnits=m  MassType=CalculateFromGeometry  InitialMassType=Specified  InitialMass=1  InitialMassUnits=kg  Density=0.001  DensityUnits=kg/m^3  SenseXLength=off  SenseYLength=off  SenseZLength=off  SenseMass=off  SenseCenterOfMass=off  SenseInertiaMatrix=off  GraphicType=FromGeometry  MarkerShape=Sphere  MarkerSize=10  GraphicVisPropType=SimpleVisualProperties  GraphicDiffuseColor=[clr1]*10/numincr+[clr2]*7/numincr  GraphicSpecularColor=[0.5 0.5 0.5 1.0]  GraphicAmbientColor=[0.15 0.15 0.15 1.0]  GraphicEmissiveColor=[0.0 0.0 0.0 1.0]  GraphicShininess=75  GraphicOpacity=1.0
      settings: AttributesFormatString=%<GraphicDiffuseColor>  SourceProductBaseCode=MS
  Variable Brick Solid8 : sm_lib/Body Elements/Variable Mass/Variable Brick Solid  XLengthType=Constant  XLength=len_x  XLengthUnits=m  YLengthType=Constant  YLength=len_y  YLengthUnits=m  ZLengthType=ProvidedByInput  ZLength=1  ZLengthUnits=m  MassType=CalculateFromGeometry  InitialMassType=Specified  InitialMass=1  InitialMassUnits=kg  Density=0.001  DensityUnits=kg/m^3  SenseXLength=off  SenseYLength=off  SenseZLength=off  SenseMass=off  SenseCenterOfMass=off  SenseInertiaMatrix=off  GraphicType=FromGeometry  MarkerShape=Sphere  MarkerSize=10  GraphicVisPropType=SimpleVisualProperties  GraphicDiffuseColor=[clr1]*9/numincr+[clr2]*8/numincr  GraphicSpecularColor=[0.5 0.5 0.5 1.0]  GraphicAmbientColor=[0.15 0.15 0.15 1.0]  GraphicEmissiveColor=[0.0 0.0 0.0 1.0]  GraphicShininess=75  GraphicOpacity=1.0
      settings: AttributesFormatString=%<GraphicDiffuseColor>  SourceProductBaseCode=MS
  Variable Brick Solid9 : sm_lib/Body Elements/Variable Mass/Variable Brick Solid  XLengthType=Constant  XLength=len_x  XLengthUnits=m  YLengthType=Constant  YLength=len_y  YLengthUnits=m  ZLengthType=ProvidedByInput  ZLength=1  ZLengthUnits=m  MassType=CalculateFromGeometry  InitialMassType=Specified  InitialMass=1  InitialMassUnits=kg  Density=0.001  DensityUnits=kg/m^3  SenseXLength=off  SenseYLength=off  SenseZLength=off  SenseMass=off  SenseCenterOfMass=off  SenseInertiaMatrix=off  GraphicType=FromGeometry  MarkerShape=Sphere  MarkerSize=10  GraphicVisPropType=SimpleVisualProperties  GraphicDiffuseColor=[clr1]*8/numincr+[clr2]*9/numincr  GraphicSpecularColor=[0.5 0.5 0.5 1.0]  GraphicAmbientColor=[0.15 0.15 0.15 1.0]  GraphicEmissiveColor=[0.0 0.0 0.0 1.0]  GraphicShininess=75  GraphicOpacity=1.0
      settings: AttributesFormatString=%<GraphicDiffuseColor>  SourceProductBaseCode=MS
  Conn1 : PMIOPort  Side=Right
  wires:
  Subsystem3/1(Out1) -> Gain/1
  Gain/1 -> Selector/1, Selector1/1, Selector2/1, Selector3/1, Selector4/1, Selector5/1, Selector6/1, Selector7/1, Selector8/1, Selector9/1, Selector10/1, Selector11/1, Selector12/1, Selector13/1, Selector14/1, Selector15/1, Selector16/1
  Selector16/1 -> Simulink-PS Converter17/1
  In1/1 -> Subsystem3/1(In1)
  Selector15/1 -> Simulink-PS Converter16/1
  Selector14/1 -> Simulink-PS Converter15/1
  Selector13/1 -> Simulink-PS Converter14/1
  Selector12/1 -> Simulink-PS Converter13/1
  Selector11/1 -> Simulink-PS Converter12/1
  Selector10/1 -> Simulink-PS Converter11/1
  Selector9/1 -> Simulink-PS Converter10/1
  Selector8/1 -> Simulink-PS Converter9/1
  Selector7/1 -> Simulink-PS Converter8/1
  Selector6/1 -> Simulink-PS Converter7/1
  Selector5/1 -> Simulink-PS Converter6/1
  Selector4/1 -> Simulink-PS Converter5/1
  Selector3/1 -> Simulink-PS Converter4/1
  Selector2/1 -> Simulink-PS Converter3/1
  Selector1/1 -> Simulink-PS Converter2/1
  Selector/1 -> Simulink-PS Converter1/1
  connections:
  Variable Brick Solid16/LConn1 -- Simulink-PS Converter17/RConn1
  Variable Brick Solid15/LConn1 -- Simulink-PS Converter16/RConn1
  Variable Brick Solid14/LConn1 -- Simulink-PS Converter15/RConn1
  Variable Brick Solid13/LConn1 -- Simulink-PS Converter14/RConn1
  Variable Brick Solid12/LConn1 -- Simulink-PS Converter13/RConn1
  Variable Brick Solid11/LConn1 -- Simulink-PS Converter12/RConn1
  Variable Brick Solid10/LConn1 -- Simulink-PS Converter11/RConn1
  Variable Brick Solid9/LConn1 -- Simulink-PS Converter10/RConn1
  Variable Brick Solid8/LConn1 -- Simulink-PS Converter9/RConn1
  Variable Brick Solid7/LConn1 -- Simulink-PS Converter8/RConn1
  Variable Brick Solid6/LConn1 -- Simulink-PS Converter7/RConn1
  Variable Brick Solid5/LConn1 -- Simulink-PS Converter6/RConn1
  Variable Brick Solid4/LConn1 -- Simulink-PS Converter5/RConn1
  Variable Brick Solid3/LConn1 -- Simulink-PS Converter4/RConn1
  Variable Brick Solid2/LConn1 -- Simulink-PS Converter3/RConn1
  Simulink-PS Converter2/RConn1 -- Variable Brick Solid1/LConn1
  Variable Brick Solid16/RConn1 -- Variable Brick Solid15/RConn1 -- Variable Brick Solid14/RConn1 -- Variable Brick Solid13/RConn1 -- Variable Brick Solid11/RConn1 -- Variable Brick Solid/RConn1 -- Conn1/RConn1 -- Variable Brick Solid4/RConn1 -- Variable Brick Solid10/RConn1 -- Variable Brick Solid9/RConn1 -- Variable Brick Solid8/RConn1 -- Variable Brick Solid7/RConn1 -- Variable Brick Solid6/RConn1 -- Variable Brick Solid5/RConn1 -- Variable Brick Solid3/RConn1 -- Variable Brick Solid2/RConn1 -- Variable Brick Solid1/RConn1 -- Variable Brick Solid12/RConn1
  Simulink-PS Converter1/RConn1 -- Variable Brick Solid/LConn1
